simulink model "Copy_2_of_PID"  (R2017a)
settings: Solver=ode5  StartTime=0.0  StopTime=15  FixedStep=0.05  MaxStep=0.05  RelTol=1e-3
libraries: simulink x2
settings Model: Creator=asus  LastModifiedBy=Lenovo

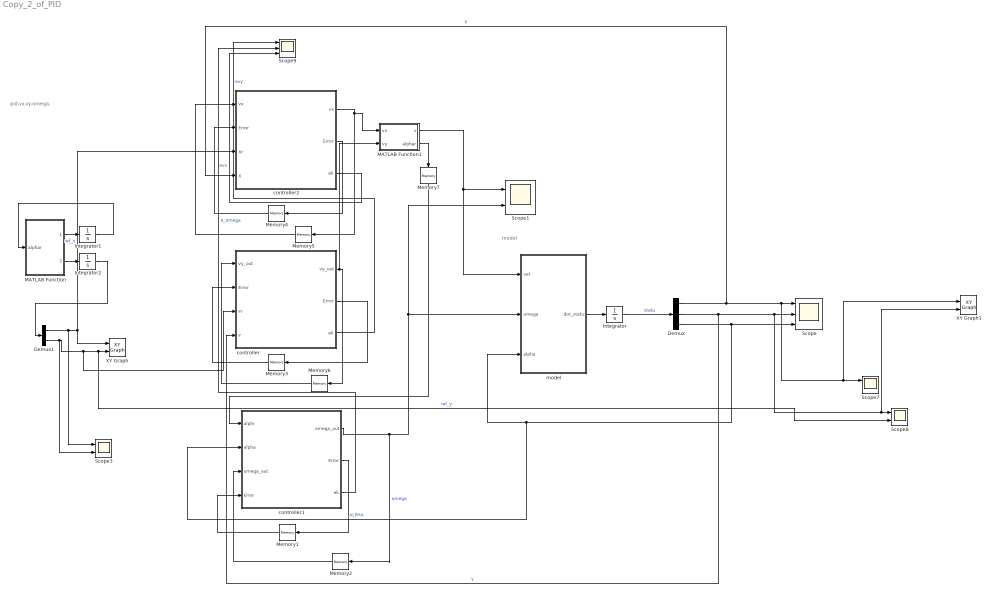
== system Copy_2_of_PID ==
  note: pid,vx,vy,omega.
  note: model
  Demux : Demux  Outputs=3
  Demux1 : Demux  Outputs=2
  Integrator : Integrator  InitialCondition=[1 -1 0 ]  IgnoreLimit=on
  Integrator1 : Integrator  InitialCondition=pi/4
  Integrator2 : Integrator
  MATLAB Function : MATLAB Function  TreatAsAtomicUnit=on
  MATLAB Function1 : MATLAB Function  TreatAsAtomicUnit=on
  Memory1 : Memory  X0=[0 0 ]
  Memory{2,5..7} (4 alike) : Memory
  Memory3 : Memory  X0=[0 0]
  Memory4 : Memory  X0=[0 0]
  Scope : Scope  NumInputPorts=3
  Scope{1,3,7..8} (4 alike) : Scope  NumInputPorts=2
  Scope9 : Scope  NumInputPorts=3
  XY Graph : simulink/Sinks/XY Graph  xmin=-10  xmax=10  ymin=-10  ymax=10  st=-1
  XY Graph1 : simulink/Sinks/XY Graph  xmin=-10  xmax=10  ymin=-10  ymax=10  st=-1
  controller : MATLAB Function  TreatAsAtomicUnit=on
  controller1 : MATLAB Function  TreatAsAtomicUnit=on
  controller2 : MATLAB Function  TreatAsAtomicUnit=on
  model : MATLAB Function  TreatAsAtomicUnit=on
  wires:
  Integrator/1 -> Demux/1  "statu"
  model/1(dot_statu) -> Integrator/1
  controller/2(Error) -> Memory3/1
  Memory3/1 -> controller/2("Error ")
  MATLAB Function/1(dot_alphar) -> Integrator1/1
  controller1/1(omega_out) -> Memory2/1, model/2(omega), Scope1/2  "omega"
  controller1/2(Error) -> Memory1/1
  Memory1/1 -> controller1/4("Error ")
  Demux/2 -> controller/4(Y), XY Graph1/2, Scope8/1, Scope/2  "Y"
  Demux/1 -> controller2/4(X), XY Graph1/1, Scope7/1, Scope/1  "X"
  MATLAB Function/2(dot_posr) -> Integrator2/1
  Demux/3 -> Scope/3, controller1/2(alpha), model/3(alpha)  "ALPHA"
  Demux1/1 -> Scope3/1, XY Graph/1, controller2/3(Xr)  "ref_x"
  Demux1/2 -> Scope3/2, controller/3(Yr), Scope8/2, XY Graph/2  "ref_y"
  Integrator1/1 -> MATLAB Function/1(alphar)
  Integrator2/1 -> Demux1/1
  controller/3(ek) -> Scope9/1  "evy"
  controller1/3(ek) -> Scope9/2  "e_omega"
  Memory2/1 -> controller1/3("omega_out ")
  controller2/2(Error) -> Memory4/1
  Memory4/1 -> controller2/2("Error ")
  controller2/1(vx) -> MATLAB Function1/1(vx), Memory5/1
  Memory5/1 -> controller2/1("vx ")
  controller2/3(ek) -> Scope9/3  "evx"
  controller/1(vy_out) -> Memory6/1, MATLAB Function1/2(vy)
  Memory6/1 -> controller/1("vy_out ")
  MATLAB Function1/1(v) -> Scope1/1, model/1(vel)
  MATLAB Function1/2(alphar) -> Memory7/1
  Memory7/1 -> controller1/1(alphr)

== matlab function Copy_2_of_PID/controller ==
  data: vy_out input; vy_out output; Error input; Error output; Yr input; Y input; ek output
function [vy_out,Error,ek] = my_vy_controller( vy_out,Error,Yr,Y)
% 程序上没有问题，在运动学模型上是可以完成任务的
% 最近修改时间：11. 20
% 基于运动学模型的   控制器
% u_out=[vx ;  omega]
% ref_vel=[xr yr alphar vr omegar]
% % e = [ex ey ealpha]
% 
% 

%% 状态量                                                                           
ek=Yr-Y;

ek_1=Error(1);
ek_2=Error(2);

kp=5;  ki=0.1;  kd=0;
delta_u=kp*(ek-ek_1)+ki*ek+kd*(ek-2*ek_1+ek_2);

vy_out=delta_u+vy_out;

ek_2=ek_1;
ek_1=ek;

Error=[ek_1;ek_2];
end



































% %% 测试是否能得到
% %    statu=[2; -2; pi/2; 0.001; 0.001; 0.001];
% %    u_out=[0; 0];
% %    ref_pos=[0;0;pi/4]; ref_vel=[2; 0; 0];  
% %    Error=[0 0 0 0];
% %% 底盘参数
% % d = 0.18;	l = 0.16;	m = 24;	Iz = 11.89;	c = 513.6; %轮胎侧偏刚度
% 
% %% 状态量                                                                           
% x = statu(1);   y = statu(2);  alpha = statu(3); 
% vx = statu(4);  vy = statu(5);    omega = statu(6);
% 
% xr=ref_pos(1);  yr=ref_pos(2);  alphar=ref_pos(3);
% vxr=ref_vel(1); vyr=ref_vel(2); omegar=ref_vel(3);
% 
% % e1k_1=Error(1); e1k_2=Error(2);
% 
% e2k_1=Error(3); e2k_2=Error(4);
%                                                                                       
% %%  误差
% ex=x-xr;    ey=y-yr;    ealpha=alpha-alphar;
% ev=vx-vxr;  eomega=omega-omegar;
% 
% e1k=ex+ey;
% % kp1=  0.4  ;   ki1= 0.4   ;   kd1=  0.4  ;
% % delta_u1=kp1*(e1k-e1k_1)+ki1*e1k+kd1*(e1k-2*e1k_1+e1k_2);
% 
% e2k=ealpha;
% kp2=0.4;  ki2=0.4;  kd2=0.4;
% delta_u2=kp2*(e2k-e2k_1)+ki2*e2k+kd2*(e2k-2*e2k_1+e2k_2);
% 
% delta_uout=[delta_u1;delta_u2];
% 
% u_out = delta_uout+u_out;
% 
% e1k_2=e1k_1;
% e1k_1=e1k;
% 
% e2k_2=e2k_1;
% e2k_1=e2k;
% 
% Error=[e1k_1;   e1k_2;   e2k_1 ;   e2k_2];
% 
% 
%

== matlab function Copy_2_of_PID/model ==
  data: vel input; dot_statu output; omega input; alpha input
function dot_statu  = model(vel,omega,alpha)



dot_alpha = omega;
dot_X=vel*cos(alpha);
dot_Y=vel*sin(alpha);



% 状态【x y alpha vx vy omega】
dot_statu = [dot_X,dot_Y,dot_alpha];

end

% max=1/wheel_radius;
% for i=1:size(wheel_omega,2)
%     if wheel_omega(i)>max
%         wheel_omega(i) = max;
%     else
%         if wheel_omega(i)<-max
%             wheel_omega(i) = -max;
%         else
%             wheel_omega(i) = wheel_omega(i);
%         end
%     end
% end

== matlab function Copy_2_of_PID/MATLAB Function ==
  data: dot_alphar output; dot_posr output; alphar input
function [dot_alphar,dot_posr] = ref(alphar)


omegar=0;

velr=1;
dot_alphar = omegar;
dot_xr=velr*cos(alphar);
dot_yr=velr*sin(alphar);

dot_posr=[dot_xr;dot_yr];

end

== matlab function Copy_2_of_PID/controller1 ==
  data: alphr input; omega_out output; alpha input; omega_out input; Error input; Error output; ek output
function [omega_out,Error,ek] = my_omega_controller(alphr,alpha, omega_out,Error)
% 程序上没有问题，在运动学模型上是可以完成任务的
% 最近修改时间：11. 20
% 基于运动学模型的   控制器
% u_out=[vx ;  omega]
% ref_vel=[xr yr alphar vr omegar]
% % e = [ex ey ealpha]
% 
%
%% 状态量                                                                           
ek=alphr-alpha;
ek_1=Error(1)
ek_2=Error(2)


% kp=0.5;  ki=0.005;  kd=0.02;
% kp=0.4;  ki=0.0000001;  kd=0;
kpx=10;  kix=0.1;  kdx=0;
% kpy=20;  kiy=0.05;  kdy=0;
delta_u=kpx*(ek-ek_1)+kix*ek+kdx*(ek-2*ek_1+ek_2);
%     kpy*(ek1-ek1_1)+kiy*ek1+kdy*(ek1-2*ek1_1+ek1_2)

omega_out=delta_u+omega_out;

ek_2=ek_1;
ek_1=ek;

Error=[ek_1;ek_2];
end



































% %% 测试是否能得到
% %    statu=[2; -2; pi/2; 0.001; 0.001; 0.001];
% %    u_out=[0; 0];
% %    ref_pos=[0;0;pi/4]; ref_vel=[2; 0; 0];  
% %    Error=[0 0 0 0];
% %% 底盘参数
% % d = 0.18;	l = 0.16;	m = 24;	Iz = 11.89;	c = 513.6; %轮胎侧偏刚度
% 
% %% 状态量                                                                           
% x = statu(1);   y = statu(2);  alpha = statu(3); 
% vx = statu(4);  vy = statu(5);    omega = statu(6);
% 
% xr=ref_pos(1);  yr=ref_pos(2);  alphar=ref_pos(3);
% vxr=ref_vel(1); vyr=ref_vel(2); omegar=ref_vel(3);
% 
% % e1k_1=Error(1); e1k_2=Error(2);
% 
% e2k_1=Error(3); e2k_2=Error(4);
%                                                                                       
% %%  误差
% ex=x-xr;    ey=y-yr;    ealpha=alpha-alphar;
% ev=vx-vxr;  eomega=omega-omegar;
% 
% e1k=ex+ey;
% % kp1=  0.4  ;   ki1= 0.4   ;   kd1=  0.4  ;
% % delta_u1=kp1*(e1k-e1k_1)+ki1*e1k+kd1*(e1k-2*e1k_1+e1k_2);
% 
% e2k=ealpha;
% kp2=0.4;  ki2=0.4;  kd2=0.4;
% delta_u2=kp2*(e2k-e2k_1)+ki2*e2k+kd2*(e2k-2*e2k_1+e2k_2);
% 
% delta_uout=[delta_u1;delta_u2];
% 
% u_out = delta_uout+u_out;
% 
% e1k_2=e1k_1;
% e1k_1=e1k;
% 
% e2k_2=e2k_1;
% e2k_1=e2k;
% 
% Error=[e1k_1;   e1k_2;   e2k_1 ;   e2k_2];
% 
% 
%

== matlab function Copy_2_of_PID/MATLAB Function1 ==
  data: vx input; v output; vy input; alphar output
function [v,alphar ]= fcn(vx,vy)

alphar=atan(vy/vx);

v = vy/sin(alphar);

== matlab function Copy_2_of_PID/controller2 ==
  data: vx output; vx input; Error input; Error output; Xr input; X input; ek output
function [vx,Error,ek] = my_vx_controller( vx,Error,Xr,X)
% 程序上没有问题，在运动学模型上是可以完成任务的
% 最近修改时间：11. 20
% 基于运动学模型的   控制器
% u_out=[vx ;  omega]
% ref_vel=[xr yr alphar vr omegar]
% % e = [ex ey ealpha]
% 
% 

%% 状态量                                                                           
ek=Xr-X;
ek_1=Error(1);
ek_2=Error(2);

kp=5;  ki=0.1;  kd=0;
delta_u=kp*(ek-ek_1)+ki*ek+kd*(ek-2*ek_1+ek_2);

vx=delta_u+vx;

ek_2=ek_1;
ek_1=ek;

Error=[ek_1;ek_2];
end



































% %% 测试是否能得到
% %    statu=[2; -2; pi/2; 0.001; 0.001; 0.001];
% %    u_out=[0; 0];
% %    ref_pos=[0;0;pi/4]; ref_vel=[2; 0; 0];  
% %    Error=[0 0 0 0];
% %% 底盘参数
% % d = 0.18;	l = 0.16;	m = 24;	Iz = 11.89;	c = 513.6; %轮胎侧偏刚度
% 
% %% 状态量                                                                           
% x = statu(1);   y = statu(2);  alpha = statu(3); 
% vx = statu(4);  vy = statu(5);    omega = statu(6);
% 
% xr=ref_pos(1);  yr=ref_pos(2);  alphar=ref_pos(3);
% vxr=ref_vel(1); vyr=ref_vel(2); omegar=ref_vel(3);
% 
% % e1k_1=Error(1); e1k_2=Error(2);
% 
% e2k_1=Error(3); e2k_2=Error(4);
%                                                                                       
% %%  误差
% ex=x-xr;    ey=y-yr;    ealpha=alpha-alphar;
% ev=vx-vxr;  eomega=omega-omegar;
% 
% e1k=ex+ey;
% % kp1=  0.4  ;   ki1= 0.4   ;   kd1=  0.4  ;
% % delta_u1=kp1*(e1k-e1k_1)+ki1*e1k+kd1*(e1k-2*e1k_1+e1k_2);
% 
% e2k=ealpha;
% kp2=0.4;  ki2=0.4;  kd2=0.4;
% delta_u2=kp2*(e2k-e2k_1)+ki2*e2k+kd2*(e2k-2*e2k_1+e2k_2);
% 
% delta_uout=[delta_u1;delta_u2];
% 
% u_out = delta_uout+u_out;
% 
% e1k_2=e1k_1;
% e1k_1=e1k;
% 
% e2k_2=e2k_1;
% e2k_1=e2k;
% 
% Error=[e1k_1;   e1k_2;   e2k_1 ;   e2k_2];
% 
% 
%
